simulink model "MSFartoystyringtask23int"  (Simulink 8.5)
settings: Solver=ode45  StartTime=tstart  StopTime=tstop  RelTol=1e-3
values from neighbouring files (symbols this model uses):
  c = 1    [run_task_2_3.m]    (also in task_2_3_int.m)
  d_1 = -0.0634    [initcontrollers.m]    (also in task_2_3_int.m)
  d_2 = 1.0463    [initcontrollers.m]    (also in task_2_3_int.m)
  delta_c_max = 25*pi/180    (= 0.436332312999)    [initcontrollers.m]    (also in task_2_3_int.m)
  K_d_heading = (2*omega_n*T-1)/K    (= -453.172205438)    [initcontrollers.m]    (also in task_2_3_int.m = -398.529411765)
  K_i_guidance = 1/300    (= 0.00333333333333)    [run_task_2_3.m]    (also in task_2_3_int.m = 6.56167979003e-06)
  K_i_heading = omega_n/10*K_p_heading    (= -0.154682779456)    [initcontrollers.m]    (also in task_2_3_int.m = -0.139294117647)
  K_i_speed = lambda^2    [initcontrollers.m]    (also in task_2_3_int.m)
  K_p_guidance = 1/delta_guidance    (= 0.00164041994751)    [task_2_3_int.m]
  K_p_heading = omega_n^2*T/K    (= -19.335347432)    [initcontrollers.m]    (also in task_2_3_int.m = -17.4117647059)
  K_p_speed = 2*lambda    [initcontrollers.m]    (also in task_2_3_int.m)
  K_windup_heading = 1    [initcontrollers.m]    (also in task_2_3_int.m)
  K_windup_speed = 2    [initcontrollers.m]    (also in task_2_3_int.m)
  m_u = 6000    [initcontrollers.m]    (also in task_2_3_int.m)
  n_c_max = 8.9    [initcontrollers.m]    (also in task_2_3_int.m)
  omega_heading = 0.05    [initcontrollers.m]    (also in task_2_3_int.m)
  omega_speed = 0.01    [initcontrollers.m]    (also in task_2_3_int.m)
  psi0 = 0    [run_task_2_3.m]    (also in task_2_3_int.m)
  r0 = 0    [run_task_2_3.m]    (also in task_2_3_int.m)
  tsamp = 10    [run_task_2_3.m]    (also in task_2_3_int.m)
  u_r_0 = 6.63    [run_task_2_3.m]    (also in task_2_3_int.m)
  v0 = [u_r_0 0]'    [run_task_2_3.m]    (also in task_2_3_int.m)
  zeta_heading = 1    [initcontrollers.m]    (also in task_2_3_int.m)
  zeta_speed = 1    [initcontrollers.m]    (also in task_2_3_int.m)
undefined symbols (not defined in the file or in its folder): headingGuidanceint, msfartoystyring, sgn
undefined symbols (not defined in the file): p0
settings Model: Creator=christh  LastModifiedBy=ONL  ExtModeAutoUpdateStatusClock=off
settings OptimizationCC: InitFltsAndDblsToZero=on
settings DebuggingCC: SolverPrmCheckMsg=warning  FcnCallInpInsideContextMsg=UseLocalSettings

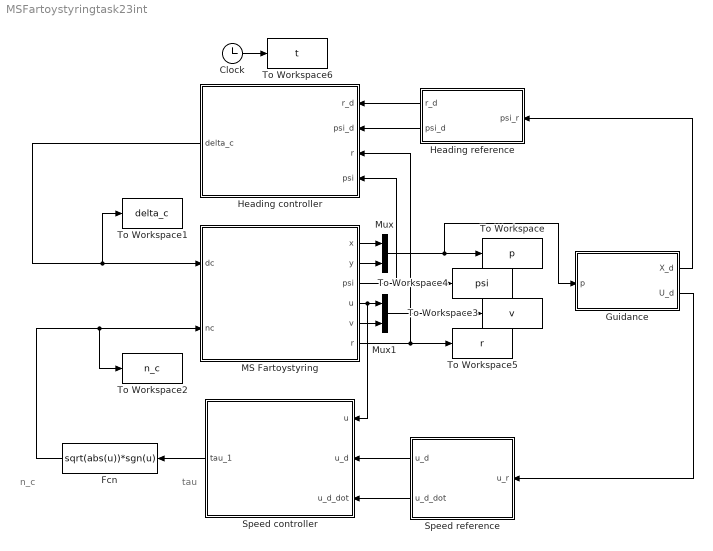
== system MSFartoystyringtask23int ==
  note: n_c
  note: tau
  Clock : Clock
  Fcn : Fcn  Expr=sqrt(abs(u))*sgn(u)
  Guidance : Subsystem
  Heading controller : Subsystem
  Heading reference : Subsystem
  MS Fartoystyring : Subsystem  mask(MS Fartoystyring for Assignment 3 G&C){x0=p0(1), y0=p0(2), u0=v0(1), v0=v0(2), psi0=psi0, r0=r0, c=c}
      mask prompts: x0 "x(t0) (m)"; y0 "y(t0) (m)"; u0 "u(t0) (m/s)"; v0 "v(t0) (m/s)"; psi0 "psi(t0) (rad)"; r0 "r(t0) (rad/s)"; c "current (0 or 1)"
      mask help:
      | Block corresponding to Figure 1 in the assignment text. Gives the response of the ship.
      |
      | The design speed of MS Fartoystyring is u=8.23 m/s.
      |
      | Input:
      | dc: commanded rudder (rad), dmax=25*pi/180
      | nc: commanded shaft speed (rad/s), nmax=85*2*pi/60
      |
      | Output:
      | x: north pos (m)
      | y: east pos (m)
      | u: surge (m/s)
      | v: sway (m/s)
      | psi: heading (rad)
      | r: yaw (rad/s)
      mask Help: Comments, bugs and help requests can be directed to the TA. Email on course website.
  Mux : Mux  Inputs=2
  Mux1 : Mux  Inputs=2
  "Speed controller " : Subsystem
  Speed reference : Subsystem
  To Workspace : ToWorkspace  VariableName=p  SampleTime=tsamp
  To Workspace1 : ToWorkspace  VariableName=delta_c  SampleTime=tsamp
  To Workspace2 : ToWorkspace  VariableName=n_c  SampleTime=tsamp
  To Workspace3 : ToWorkspace  VariableName=v  SampleTime=tsamp
  To Workspace4 : ToWorkspace  VariableName=psi  SampleTime=tsamp
  To Workspace5 : ToWorkspace  VariableName=r  SampleTime=tsamp
  To Workspace6 : ToWorkspace  VariableName=t  SampleTime=tsamp
  wires:
  Clock/1 -> To Workspace6/1
  MS Fartoystyring/1(x) -> Mux/1
  MS Fartoystyring/2(y) -> Mux/2
  MS Fartoystyring/5(v) -> Mux1/2
  Mux/1 -> Guidance/1(p), To Workspace/1
  Mux1/1 -> To Workspace3/1
  MS Fartoystyring/3(psi) -> Heading controller/4(psi), To Workspace4/1
  MS Fartoystyring/6(r) -> Heading controller/3(r), To Workspace5/1
  Heading controller/1(delta_c) -> To Workspace1/1, MS Fartoystyring/1(dc)
  Heading reference/1(r_d) -> Heading controller/1("r_d ")
  MS Fartoystyring/4(u) -> "Speed controller "/1(u), Mux1/1
  "Speed controller "/1(tau_1) -> Fcn/1
  Fcn/1 -> To Workspace2/1, MS Fartoystyring/2(nc)
  Speed reference/1(u_d) -> "Speed controller "/2(u_d)
  Speed reference/2(u_d_dot) -> "Speed controller "/3(u_d_dot)
  Heading reference/2(psi_d) -> Heading controller/2("psi_d ")
  Guidance/2(U_d) -> Speed reference/1(u_r)
  Guidance/1(X_d) -> Heading reference/1(psi_r)

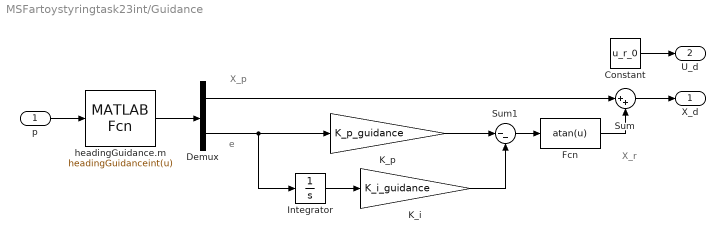
== system MSFartoystyringtask23int/Guidance ==
  note: e
  note: X_r
  note: X_p
  p : Inport
  Constant : Constant  Value=u_r_0
  Demux : Demux  Outputs=2
  Fcn : Fcn  Expr=atan(u)
  Integrator : Integrator
  "K_i " : Gain  Gain=K_i_guidance
  K_p : Gain  Gain=K_p_guidance
  Sum : Sum  Inputs=|++
  Sum1 : Sum  Inputs=|--
  "headingGuidance.m " : MATLABFcn  MATLABFcn=headingGuidanceint(u)  OutputDimensions=2
  X_d : Outport
  U_d : Outport  Port=2
  wires:
  p/1 -> "headingGuidance.m "/1
  "headingGuidance.m "/1 -> Demux/1
  Demux/1 -> Sum/1
  Integrator/1 -> "K_i "/1
  Demux/2 -> K_p/1, Integrator/1
  "K_i "/1 -> Sum1/2
  Sum1/1 -> Fcn/1
  Fcn/1 -> Sum/2
  K_p/1 -> Sum1/1
  Sum/1 -> X_d/1
  Constant/1 -> U_d/1

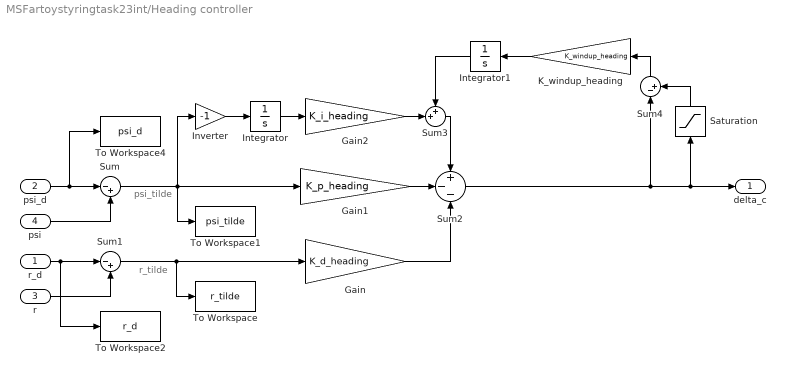
== system MSFartoystyringtask23int/Heading controller ==
  note: r_tilde
  note: psi_tilde
  "r_d " : Inport
  "psi_d " : Inport  Port=2
  r : Inport  Port=3
  psi : Inport  Port=4
  Gain : Gain  Gain=K_d_heading
  Gain1 : Gain  Gain=K_p_heading
  Gain2 : Gain  Gain=K_i_heading
  Integrator : Integrator
  Integrator1 : Integrator
  Inverter : Gain  Gain=-1
  "K_windup_heading " : Gain  Gain=K_windup_heading
  Saturation : Saturate  UpperLimit=delta_c_max  LowerLimit=-delta_c_max
  Sum : Sum  Inputs=|-+
  Sum1 : Sum  Inputs=|-+
  Sum2 : Sum  Inputs=+--
  Sum3 : Sum  Inputs=++|
  Sum4 : Sum  Inputs=|-+
  To Workspace : ToWorkspace  VariableName=r_tilde  SampleTime=tsamp
  To Workspace1 : ToWorkspace  VariableName=psi_tilde  SampleTime=tsamp
  To Workspace2 : ToWorkspace  VariableName=r_d  SampleTime=tsamp
  To Workspace4 : ToWorkspace  VariableName=psi_d  SampleTime=tsamp
  delta_c : Outport
  wires:
  Sum1/1 -> To Workspace/1, Gain/1
  Sum/1 -> Inverter/1, To Workspace1/1, Gain1/1
  Sum2/1 -> Sum4/1, Saturation/1, delta_c/1
  Gain1/1 -> Sum2/2
  Gain/1 -> Sum2/3
  Integrator/1 -> Gain2/1
  "r_d "/1 -> To Workspace2/1, Sum1/1
  r/1 -> Sum1/2
  psi/1 -> Sum/2
  "psi_d "/1 -> To Workspace4/1, Sum/1
  "K_windup_heading "/1 -> Integrator1/1
  Gain2/1 -> Sum3/2
  Integrator1/1 -> Sum3/1
  Sum3/1 -> Sum2/1
  Saturation/1 -> Sum4/2
  Sum4/1 -> "K_windup_heading "/1
  Inverter/1 -> Integrator/1

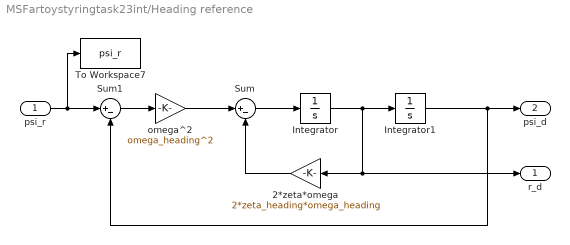
== system MSFartoystyringtask23int/Heading reference ==
  psi_r : Inport
  2*zeta*omega : Gain  Gain=2*zeta_heading*omega_heading
  Integrator : Integrator  InitialCondition=r0
  Integrator1 : Integrator  InitialCondition=psi0
  Sum : Sum  Inputs=|+-
  Sum1 : Sum  Inputs=|+-
  To Workspace7 : ToWorkspace  VariableName=psi_r  SampleTime=tsamp
  omega^2 : Gain  Gain=omega_heading^2
  r_d : Outport
  psi_d : Outport  Port=2
  wires:
  Integrator/1 -> 2*zeta*omega/1, r_d/1, Integrator1/1
  omega^2/1 -> Sum/1
  Sum/1 -> Integrator/1
  psi_r/1 -> Sum1/1, To Workspace7/1
  Sum1/1 -> omega^2/1
  Integrator1/1 -> psi_d/1, Sum1/2
  2*zeta*omega/1 -> Sum/2

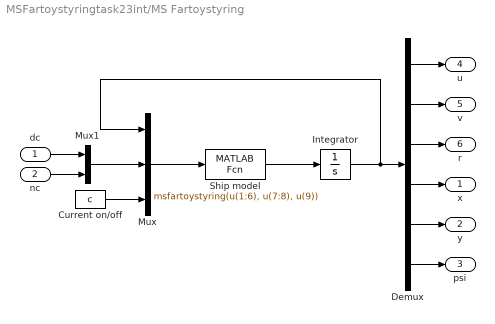
== system MSFartoystyringtask23int/MS Fartoystyring ==
  dc : Inport
  nc : Inport  Port=2
  Current on/off : Constant  Value=c
  Demux : Demux  Outputs=6
  Integrator : Integrator  InitialCondition=[u0 v0 r0 x0 y0 psi0]'
  Mux : Mux  Inputs=3
  Mux1 : Mux  Inputs=2
  Ship model : MATLABFcn  MATLABFcn=msfartoystyring(u(1:6), u(7:8), u(9))  OutputDimensions=6
  x : Outport
  y : Outport  Port=2
  psi : Outport  Port=3
  u : Outport  Port=4
  v : Outport  Port=5
  r : Outport  Port=6
  wires:
  Integrator/1 -> Mux/1, Demux/1
  Mux1/1 -> Mux/2
  dc/1 -> Mux1/1
  nc/1 -> Mux1/2
  Demux/1 -> u/1
  Demux/2 -> v/1
  Demux/3 -> r/1
  Demux/4 -> x/1
  Demux/5 -> y/1
  Demux/6 -> psi/1
  Current on/off/1 -> Mux/3
  Ship model/1 -> Integrator/1
  Mux/1 -> Ship model/1

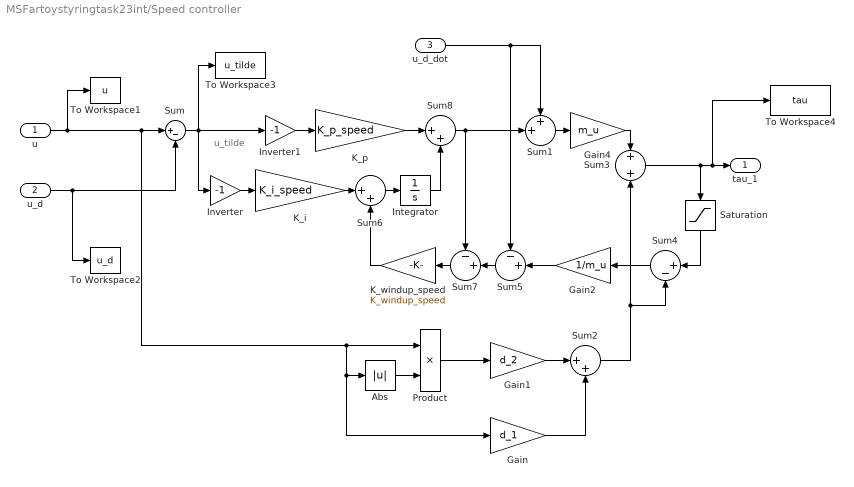
== system MSFartoystyringtask23int/Speed controller  ==
  note: u_tilde
  u : Inport
  u_d : Inport  Port=2
  u_d_dot : Inport  Port=3
  Abs : Abs
  Gain : Gain  Gain=d_1
  Gain1 : Gain  Gain=d_2
  Gain2 : Gain  Gain=1/m_u
  Gain4 : Gain  Gain=m_u
  Integrator : Integrator
  Inverter : Gain  Gain=-1
  Inverter1 : Gain  Gain=-1
  "K_i " : Gain  Gain=K_i_speed
  K_p : Gain  Gain=K_p_speed
  K_windup_speed : Gain  Gain=K_windup_speed
  Product : Product
  Saturation : Saturate  UpperLimit=n_c_max^2  LowerLimit=-n_c_max^2
  Sum : Sum  Inputs=|+-
  Sum1 : Sum  Inputs=++|
  Sum2 : Sum  Inputs=|++
  Sum3 : Sum
  Sum4 : Sum  Inputs=|+-
  Sum5 : Sum  Inputs=-+|
  Sum6 : Sum  Inputs=|++
  Sum7 : Sum  Inputs=-+|
  Sum8 : Sum  Inputs=|++
  To Workspace1 : ToWorkspace  VariableName=u  SampleTime=tsamp
  To Workspace2 : ToWorkspace  VariableName=u_d  SampleTime=tsamp
  To Workspace3 : ToWorkspace  VariableName=u_tilde  SampleTime=tsamp
  To Workspace4 : ToWorkspace  VariableName=tau  SampleTime=tsamp
  tau_1 : Outport
  wires:
  u/1 -> To Workspace1/1, Gain/1, Abs/1, Product/1, Sum/1
  u_d/1 -> To Workspace2/1, Sum/2
  Sum/1 -> To Workspace3/1, Inverter1/1, Inverter/1
  K_p/1 -> Sum8/1
  Gain1/1 -> Sum2/1
  Product/1 -> Gain1/1
  Abs/1 -> Product/2
  Gain/1 -> Sum2/2
  Inverter/1 -> "K_i "/1
  Gain4/1 -> Sum3/1
  Sum2/1 -> Sum3/2, Sum4/2
  Saturation/1 -> Sum4/1
  Sum4/1 -> Gain2/1
  Gain2/1 -> Sum5/2
  Integrator/1 -> Sum8/2
  "K_i "/1 -> Sum6/1
  Sum6/1 -> Integrator/1
  K_windup_speed/1 -> Sum6/2
  Sum8/1 -> Sum1/2, Sum7/1
  Sum1/1 -> Gain4/1
  u_d_dot/1 -> Sum1/1, Sum5/1
  Sum3/1 -> Saturation/1, To Workspace4/1, tau_1/1
  Inverter1/1 -> K_p/1
  Sum7/1 -> K_windup_speed/1
  Sum5/1 -> Sum7/2

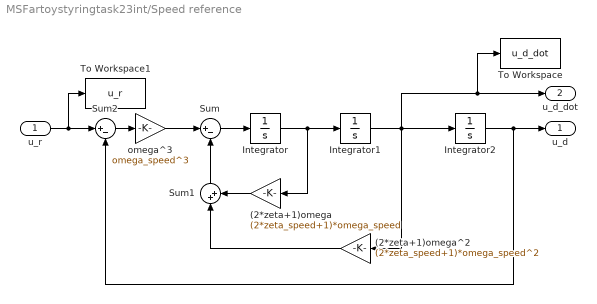
== system MSFartoystyringtask23int/Speed reference ==
  u_r : Inport
  (2*zeta+1)omega : Gain  Gain=(2*zeta_speed+1)*omega_speed
  (2*zeta+1)omega^2 : Gain  Gain=(2*zeta_speed+1)*omega_speed^2
  Integrator : Integrator
  Integrator1 : Integrator
  Integrator2 : Integrator  InitialCondition=u_r_0
  Sum : Sum  Inputs=|+-
  Sum1 : Sum  Inputs=|++
  Sum2 : Sum  Inputs=|+-
  To Workspace : ToWorkspace  VariableName=u_d_dot  SampleTime=tsamp
  To Workspace1 : ToWorkspace  VariableName=u_r  SampleTime=tsamp
  omega^3 : Gain  Gain=omega_speed^3
  u_d : Outport
  u_d_dot : Outport  Port=2
  wires:
  Integrator2/1 -> Sum2/2, u_d/1
  Integrator/1 -> Integrator1/1, (2*zeta+1)omega/1
  Integrator1/1 -> (2*zeta+1)omega^2/1, To Workspace/1, u_d_dot/1, Integrator2/1
  omega^3/1 -> Sum/1
  Sum/1 -> Integrator/1
  Sum1/1 -> Sum/2
  (2*zeta+1)omega^2/1 -> Sum1/1
  (2*zeta+1)omega/1 -> Sum1/2
  Sum2/1 -> omega^3/1
  u_r/1 -> To Workspace1/1, Sum2/1
